simulink model "Time_Delayed_Controller_fixed"  (R2024b)
settings: Solver=VariableStepAuto  StartTime=0.0  StopTime=5  FixedStep=0.001  RelTol=1e-3
undefined symbols (not defined in the file): q_goal_rad, q_start
libraries: robotmaniplib x1, robotcorelib x1
settings Model: Creator=변재형  LastModifiedBy=변재형

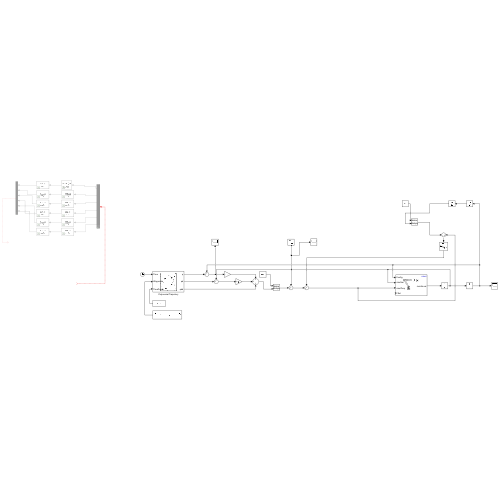
[thumbnail: Simulink's stored preview of the top-level diagram]
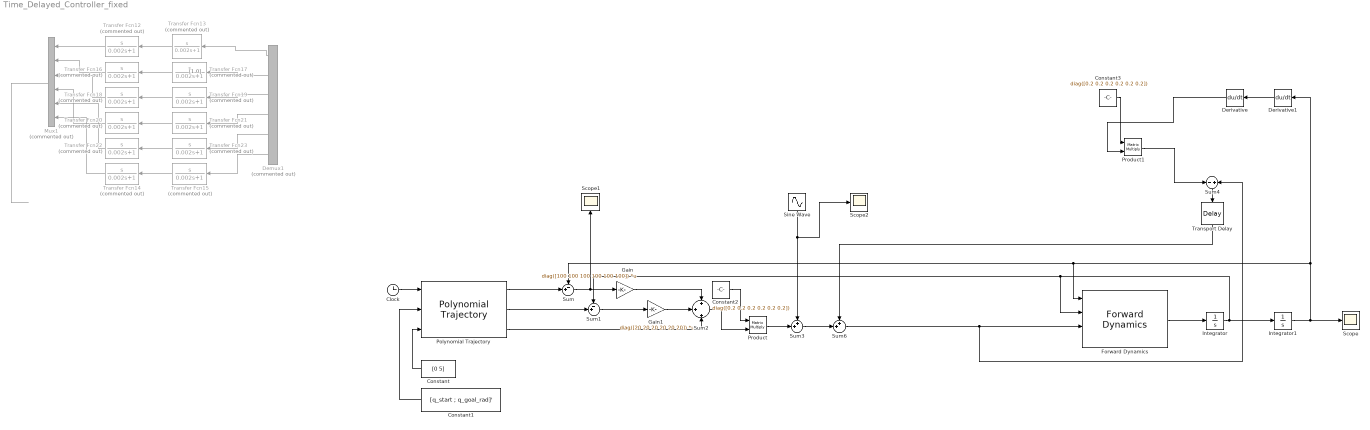
== system Time_Delayed_Controller_fixed ==
  note: [1 0]
  Clock : Clock
      settings: Decimation=5
  Constant : Constant  Value=[0 5]
  Constant1 : Constant  Value=[q_start ; q_goal_rad]'
  Constant2 : Constant  Value=diag([0.2 0.2 0.2 0.2 0.2 0.2])
  Constant3 : Constant  Value=diag([0.2 0.2 0.2 0.2 0.2 0.2])
  Demux1 : Demux  Commented=on  Outputs=6
  Derivative : Derivative
  Derivative1 : Derivative
  Forward Dynamics : robotmaniplib/Forward Dynamics  RigidBodyTree=robot  SimulateUsing=Interpreted execution
  Gain : Gain  Gain=diag([100 100 100 100 100 100])  Multiplication=Matrix(K*u)
  Gain1 : Gain  Gain=diag([20 20 20 20 20 20])  Multiplication=Matrix(K*u)
  Integrator : Integrator
  Integrator1 : Integrator
  Mux1 : Mux  Commented=on  Inputs=6
  Polynomial Trajectory : robotcorelib/Polynomial Trajectory  WaypointSource=External  Waypoints=[ 0, 2, 1, 5, 0; -1, 3, 1, 4, 4 ]  TimePoints=[ 0, 1, 2, 3, 4 ]  TimeInterval=[ 1, 4 ]  Method=Quintic Polynomial  ParameterSource=Internal  VelocityBoundaryCondition=zeros( 6, 2 )  AccelerationBoundaryCondition=zeros( 6, 2 )  SimulateUsing=Interpreted execution
  Product : Product  Multiplication=Matrix(*)
  Product1 : Product  Multiplication=Matrix(*)
  Scope : Scope
  Scope1 : Scope
  Scope2 : Scope
  Sine Wave : Sin  Amplitude=0.1  Frequency=10  SampleTime=0
  Sum : Sum  Inputs=-+|
  Sum1 : Sum  Inputs=-+|
  Sum2 : Sum  Inputs=+|+|+
  Sum3 : Sum  Inputs=++|
  Sum4 : Sum  Inputs=-|+
  Sum6 : Sum  Inputs=++|
  Transfer Fcn{12..23} (12 alike) : TransferFcn  Commented=on  Numerator=[1 0]  Denominator=[0.002 1]
  Transport Delay : TransportDelay  DelayTime=0.001  BufferSize=5000
  wires:
  Constant/1 -> Polynomial Trajectory/3
  Constant1/1 -> Polynomial Trajectory/2
  Clock/1 -> Polynomial Trajectory/1
  Integrator/1 -> Forward Dynamics/2, Sum1/1, Integrator1/1
  Polynomial Trajectory/1 -> Sum/2
  Sum/1 -> Scope1/1, Gain/1
  Polynomial Trajectory/2 -> Sum1/2
  Sum1/1 -> Gain1/1
  Gain1/1 -> Sum2/2
  Gain/1 -> Sum2/1
  Polynomial Trajectory/3 -> Sum2/3
  Sum2/1 -> Product/2
  Integrator1/1 -> Derivative1/1, Sum/1, Forward Dynamics/1, Scope/1
  Demux1/3 -> Transfer Fcn19/1
  Transfer Fcn17/1 -> Transfer Fcn16/1
  Demux1/2 -> Transfer Fcn17/1
  Demux1/5 -> Transfer Fcn23/1
  Transfer Fcn18/1 -> Mux1/3
  Transfer Fcn16/1 -> Mux1/2
  Transfer Fcn12/1 -> Mux1/1
  ? -> Demux1/1
  Transfer Fcn15/1 -> Transfer Fcn14/1
  Transfer Fcn13/1 -> Transfer Fcn12/1
  Demux1/1 -> Transfer Fcn13/1
  Demux1/6 -> Transfer Fcn15/1
  Demux1/4 -> Transfer Fcn21/1
  Transfer Fcn14/1 -> Mux1/6
  Transfer Fcn22/1 -> Mux1/5
  Transfer Fcn23/1 -> Transfer Fcn22/1
  Transfer Fcn19/1 -> Transfer Fcn18/1
  Transfer Fcn21/1 -> Transfer Fcn20/1
  Mux1/1 -> ?
  Transfer Fcn20/1 -> Mux1/4
  Forward Dynamics/1 -> Integrator/1
  Product/1 -> Sum3/2
  Sine Wave/1 -> Sum3/1, Scope2/1
  Sum6/1 -> Sum4/2, Forward Dynamics/3
  Constant2/1 -> Product/1
  Derivative1/1 -> Derivative/1
  Sum3/1 -> Sum6/2
  Constant3/1 -> Product1/1
  Derivative/1 -> Product1/2
  Product1/1 -> Sum4/1
  Sum4/1 -> Transport Delay/1
  Transport Delay/1 -> Sum6/1
